simulink model "Precision_Stability_Transient"  (R2012b)
settings: Solver=ode15s  StartTime=0.0  StopTime=30.0  RelTol=1e-3
libraries: slctrlblks x1, simulink x1
settings Model: Creator=Viktor  LastModifiedBy=Viktor

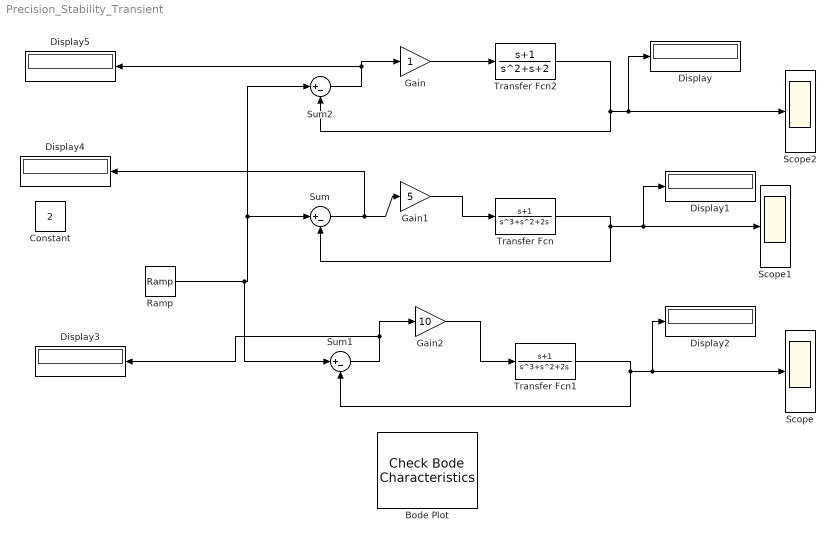
== system Precision_Stability_Transient ==
  Bode Plot : slctrlblks/Model Verification/Check Bode  Characteristics  InstantiateOnLoad=on  LinearizationIOs={'/Gain', 1, 'in', 'off', '';'/Transfer Fcn2', 1, 'out', 'off', ''}  LinearizeAt=SnapshotTimes  SnapshotTimes=[0]  TriggerType=rising  SampleTime=auto  RateConversionMethod=zoh  PreWarpFreq=10  UseExactDelayModel=off  UseFullBlockNameLabels=off  UseBusSignalLabels=off  enabled=on  stopWhenAssertionFail=off  export=off  ViewDlgPos=[1 41 1366 652]  OpenViewOnLoad=off  LaunchViewOnOpen=off  FrequencyUnits=rad/s  MagnitudeUnits=dB  PhaseUnits=deg  TimeUnits=seconds  EnableUpperBound=off  UpperBoundFrequencies=[]  UpperBoundMagnitudes=[]  EnableLowerBound=off  LowerBoundFrequencies=[]  LowerBoundMagnitudes=[]
  Constant : Constant  Value=2
  Display{,1..5} (6 alike) : Display
  Gain : Gain
  Gain1 : Gain  Gain=5
  Gain2 : Gain  Gain=10
  Ramp : simulink/Sources/Ramp  slope=2  start=0  X0=0
  Scope : Scope
  Scope1 : Scope
  Scope2 : Scope
      settings: SaveName=ScopeData2
  Sum : Sum  Inputs=|+-
  Sum1 : Sum  Inputs=|+-
  Sum2 : Sum  Inputs=|+-
  Transfer Fcn : TransferFcn  Numerator=[1 1]  Denominator=[1 1 2 0]
  Transfer Fcn1 : TransferFcn  Numerator=[1 1]  Denominator=[1 1 2 0]
  Transfer Fcn2 : TransferFcn  Numerator=[1 1]  Denominator=[1 1 2 ]
  wires:
  Gain1/1 -> Transfer Fcn/1
  Transfer Fcn/1 -> Sum/2, Display1/1, Scope1/1
  Sum/1 -> Gain1/1, Display4/1
  Gain2/1 -> Transfer Fcn1/1
  Transfer Fcn1/1 -> Display2/1, Scope/1, Sum1/2
  Gain/1 -> Transfer Fcn2/1
  Transfer Fcn2/1 -> Display/1, Scope2/1, Sum2/2
  Sum2/1 -> Gain/1, Display5/1
  Sum1/1 -> Gain2/1, Display3/1
  Ramp/1 -> Sum1/1, Sum/1, Sum2/1
